simulink model "lpv_modeling_compact"  (R2022b)
settings: Solver=VariableStepAuto  StartTime=0.0  StopTime=25  RelTol=1e-3
values from neighbouring files (symbols this model uses):
  B = [0;0;1]    [coop_lpv.m]    (also in graph_def.m = [1;1;1;1]; lpv_cooperative_control_auto.m; lpv_cooperative_control_man.m)
  C = [1 1 1]    [coop_lpv.m]    (also in lpv_cooperative_control_auto.m; lpv_cooperative_control_man.m)
  D = [0 ;0; 0]    [coop_lpv.m]    (also in graph_def.m = diag(L0); lpv_cooperative_control_auto.m = [0;0;0]; lpv_cooperative_control_man.m = [0;0;0])
  K0 = value(Y0)*inv(value(X))    [lpv_cooperative_control_auto.m]    (also in lpv_cooperative_control_man.m = K_max + theta_max/(theta_max - theta_min)*K_min - theta_max/)
  K1 = value(Y1)*inv(value(X))    [lpv_cooperative_control_auto.m]    (also in lpv_cooperative_control_man.m = K_max/(theta_max - theta_min) - K_min/(theta_max - theta_min)
libraries: cstblocks x4
settings Model: Creator=phatdo  LastModifiedBy=phatdo

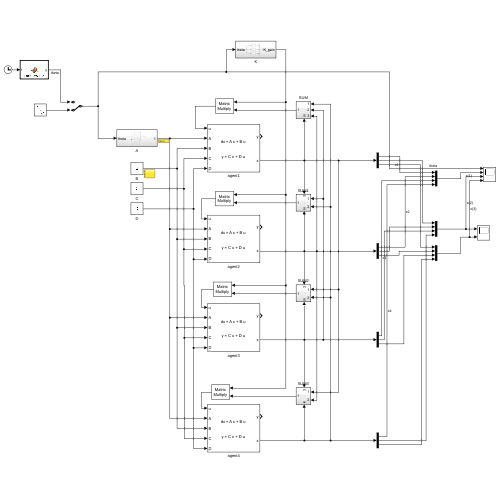
[thumbnail: Simulink's stored preview of the top-level diagram]
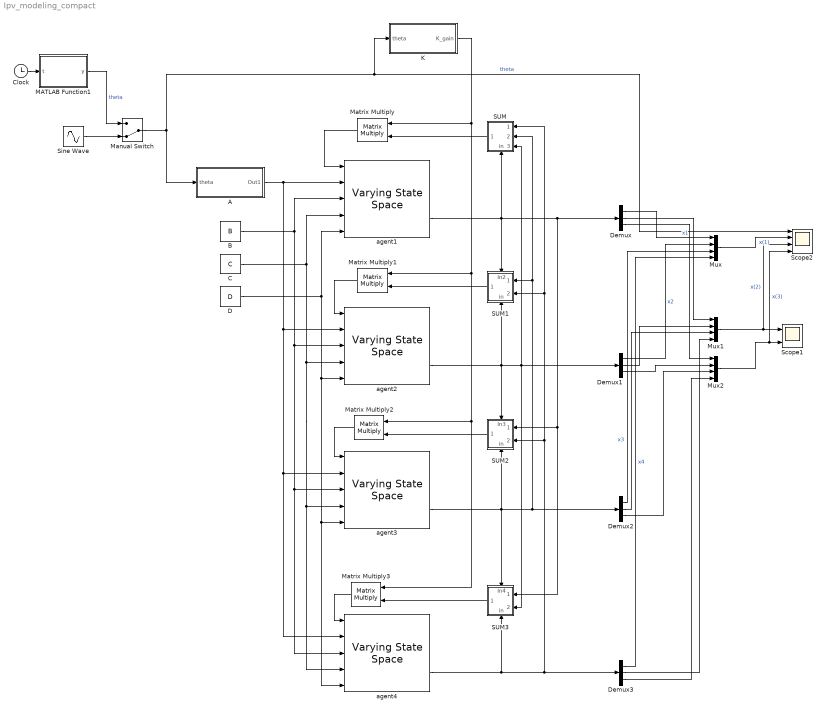
== system lpv_modeling_compact ==
  A : Subsystem
  B : Constant  Value=B
  C : Constant  Value=C  VectorParams1D=off
  Clock : Clock
  D : Constant  Value=D  VectorParams1D=off
  Demux{,1..3} (4 alike) : Demux  Outputs=3
  K : Subsystem
  MATLAB Function1 : MATLAB Function  TreatAsAtomicUnit=on
  Manual Switch : ManualSwitch  CurrentSetting=0
  Matrix Multiply{,1..3} (4 alike) : Product  Multiplication=Matrix(*)
  Mux : Mux
  Mux1 : Mux
  Mux2 : Mux
  SUM : Subsystem
      settings: PortSchema="{\"entries\":[{\"content\":{\"sides\":[{\"content\":{\"connectorIds\":[\"In1\",\"In2\",\"In3\"]},\"type\":\"ConnectorPlacement.EquallySpacedRectSide\",\"uuid\":\"fd34f642-52c8-46e7-b483-8376a438fe66\"},{\"content\":{\"connectorIds\":[\"Out1\"],\"side\":\"RIGHT\"},\"type\":\"ConnectorPlacement.EquallySpacedRectSide\",\"uuid\":\"dec59217-61bd-4aab-963d-2963be1a00c7\"},{\"content\":{\"connectorIds\":[],\"side\":\"TOP\"},\"type\":\"ConnectorPlacement.EquallySpacedRectSide\",\"uuid\":\"ad186b4c-cbd3-48c5-96df-e457cdb7fc4b\"},{\"content\":{\"connectorIds\":[\"In4\"],\"side\":\"BOTTOM\"},\"type\":\"ConnectorPlacement.EquallySpacedRectSide\",\"uuid\":\"5c94262a-f8a6-490c-bbcf-ff9d903d64fd\"}]},\"type\":\"ConnectorPlacement.EquallySpacedConnector\",\"uuid\":\"0cd37f9c-6610-4f40-8695-26be4f4b0f20\"}],\"packageUris\":[\"http://schema.mathworks.com/mf0/Connector/R2020b\"],\"version\":\"1.0\"}"
  SUM1 : Subsystem
      settings: PortSchema="{\"entries\":[{\"content\":{\"sides\":[{\"content\":{\"connectorIds\":[\"In1\",\"In2\"]},\"type\":\"ConnectorPlacement.EquallySpacedRectSide\",\"uuid\":\"fd34f642-52c8-46e7-b483-8376a438fe66\"},{\"content\":{\"connectorIds\":[\"Out1\"],\"side\":\"RIGHT\"},\"type\":\"ConnectorPlacement.EquallySpacedRectSide\",\"uuid\":\"dec59217-61bd-4aab-963d-2963be1a00c7\"},{\"content\":{\"connectorIds\":[\"In3\"],\"side\":\"TOP\"},\"type\":\"ConnectorPlacement.EquallySpacedRectSide\",\"uuid\":\"ad186b4c-cbd3-48c5-96df-e457cdb7fc4b\"},{\"content\":{\"connectorIds\":[\"In4\"],\"side\":\"BOTTOM\"},\"type\":\"ConnectorPlacement.EquallySpacedRectSide\",\"uuid\":\"67af91ab-fe79-430a-80ec-5e8b5dd21872\"}]},\"type\":\"ConnectorPlacement.EquallySpacedConnector\",\"uuid\":\"0cd37f9c-6610-4f40-8695-26be4f4b0f20\"}],\"packageUris\":[\"http://schema.mathworks.com/mf0/Connector/R2020b\"],\"version\":\"1.0\"}"
  SUM2 : Subsystem
      settings: PortSchema="{\"entries\":[{\"content\":{\"sides\":[{\"content\":{\"connectorIds\":[\"In1\",\"In2\"]},\"type\":\"ConnectorPlacement.EquallySpacedRectSide\",\"uuid\":\"fd34f642-52c8-46e7-b483-8376a438fe66\"},{\"content\":{\"connectorIds\":[\"Out1\"],\"side\":\"RIGHT\"},\"type\":\"ConnectorPlacement.EquallySpacedRectSide\",\"uuid\":\"dec59217-61bd-4aab-963d-2963be1a00c7\"},{\"content\":{\"connectorIds\":[\"In3\"],\"side\":\"TOP\"},\"type\":\"ConnectorPlacement.EquallySpacedRectSide\",\"uuid\":\"ad186b4c-cbd3-48c5-96df-e457cdb7fc4b\"},{\"content\":{\"connectorIds\":[\"In4\"],\"side\":\"BOTTOM\"},\"type\":\"ConnectorPlacement.EquallySpacedRectSide\",\"uuid\":\"5210531a-3471-4c70-b5b2-3cd9230d9329\"}]},\"type\":\"ConnectorPlacement.EquallySpacedConnector\",\"uuid\":\"0cd37f9c-6610-4f40-8695-26be4f4b0f20\"}],\"packageUris\":[\"http://schema.mathworks.com/mf0/Connector/R2020b\"],\"version\":\"1.0\"}"
  SUM3 : Subsystem
      settings: PortSchema="{\"entries\":[{\"content\":{\"sides\":[{\"content\":{\"connectorIds\":[\"In1\",\"In2\"]},\"type\":\"ConnectorPlacement.EquallySpacedRectSide\",\"uuid\":\"fd34f642-52c8-46e7-b483-8376a438fe66\"},{\"content\":{\"connectorIds\":[\"Out1\"],\"side\":\"RIGHT\"},\"type\":\"ConnectorPlacement.EquallySpacedRectSide\",\"uuid\":\"dec59217-61bd-4aab-963d-2963be1a00c7\"},{\"content\":{\"connectorIds\":[\"In3\"],\"side\":\"TOP\"},\"type\":\"ConnectorPlacement.EquallySpacedRectSide\",\"uuid\":\"ad186b4c-cbd3-48c5-96df-e457cdb7fc4b\"},{\"content\":{\"connectorIds\":[\"In4\"],\"side\":\"BOTTOM\"},\"type\":\"ConnectorPlacement.EquallySpacedRectSide\",\"uuid\":\"2ed431c9-bcc5-48d0-b09c-89e6b317baf5\"}]},\"type\":\"ConnectorPlacement.EquallySpacedConnector\",\"uuid\":\"0cd37f9c-6610-4f40-8695-26be4f4b0f20\"}],\"packageUris\":[\"http://schema.mathworks.com/mf0/Connector/R2020b\"],\"version\":\"1.0\"}"
  Scope1 : Scope  NumInputPorts=2
  Scope2 : Scope  NumInputPorts=4
  Sine Wave : Sin  Amplitude=0.5  SampleTime=0
  agent1 : cstblocks/Linear Parameter Varying/Varying State Space  x0=[2;0;0]  xNames=''  OutputX=on  OutputDX=off
  agent2 : cstblocks/Linear Parameter Varying/Varying State Space  x0=[0.5;0;0]  xNames=''  OutputX=on  OutputDX=off
  agent3 : cstblocks/Linear Parameter Varying/Varying State Space  x0=[-0.2;0;0]  xNames=''  OutputX=on  OutputDX=off
  agent4 : cstblocks/Linear Parameter Varying/Varying State Space  x0=[-1.8;0;0]  xNames=''  OutputX=on  OutputDX=off
  wires:
  Clock/1 -> MATLAB Function1/1(t)
  Manual Switch/1 -> Scope2/1, K/1(theta), A/1(theta)  "theta"
  C/1 -> agent4/4, agent3/4, agent2/4, agent1/4
  B/1 -> agent4/3, agent3/3, agent2/3, agent1/3
  D/1 -> agent1/5, agent4/5, agent3/5, agent2/5
  A/1(Out1) -> agent4/2, agent3/2, agent2/2, agent1/2
  Matrix Multiply/1 -> agent1/1
  Matrix Multiply1/1 -> agent2/1
  Matrix Multiply2/1 -> agent3/1
  Matrix Multiply3/1 -> agent4/1
  Demux/1 -> Mux/1  "x1"
  Demux1/1 -> Mux/2  "x2"
  Demux2/1 -> Mux/3  "x3"
  Demux3/1 -> Mux/4  "x4"
  Mux/1 -> Scope2/2  "x(1)"
  SUM/1(Out1) -> Matrix Multiply/2
  SUM1/1(Out1) -> Matrix Multiply1/2
  SUM2/1(Out1) -> Matrix Multiply2/2
  SUM3/1(Out1) -> Matrix Multiply3/2
  K/1(K_gain) -> Matrix Multiply/1, Matrix Multiply1/1, Matrix Multiply2/1, Matrix Multiply3/1
  agent1/2 -> SUM2/1(In2), SUM3/1(In2), Demux/1, SUM1/3(In2), SUM/4(in)
  agent2/2 -> SUM/3(In2), Demux1/1, SUM3/2(In3), SUM2/3(In3), SUM1/4(in)
  agent3/2 -> SUM1/1(In4), SUM/2(In4), Demux2/1, SUM3/3(In4), SUM2/4(in)
  agent4/2 -> SUM3/4(in), SUM2/2(In4), SUM1/2(In3), SUM/1(In3), Demux3/1
  MATLAB Function1/1(y) -> Manual Switch/1  "theta"
  Sine Wave/1 -> Manual Switch/2
  Demux/2 -> Mux1/1
  Demux1/2 -> Mux1/2
  Demux2/2 -> Mux1/3
  Demux3/2 -> Mux1/4
  Mux1/1 -> Scope2/3, Scope1/1  "x(2)"
  Demux/3 -> Mux2/1
  Demux1/3 -> Mux2/2
  Demux2/3 -> Mux2/3
  Demux3/3 -> Mux2/4
  Mux2/1 -> Scope2/4, Scope1/2  "x(3)"

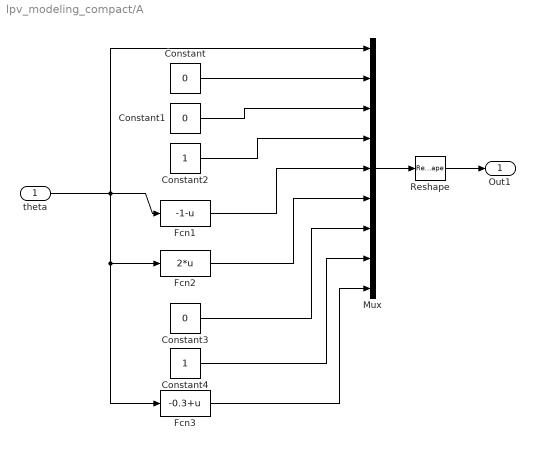
== system lpv_modeling_compact/A ==
  theta : Inport
  Constant : Constant  Value=0
  Constant1 : Constant  Value=0
  Constant2 : Constant
  Constant3 : Constant  Value=0
  Constant4 : Constant
  Fcn1 : Fcn  Expr=-1-u
  Fcn2 : Fcn  Expr=2*u
  Fcn3 : Fcn  Expr=-0.3+u
  Mux : Mux  Inputs=9
  Reshape : Reshape  OutputDimensionality=Customize  OutputDimensions=[3,3]
  Out1 : Outport
  wires:
  Mux/1 -> Reshape/1
  theta/1 -> Fcn3/1, Fcn2/1, Fcn1/1, Mux/1
  Constant/1 -> Mux/2
  Constant1/1 -> Mux/3
  Constant2/1 -> Mux/4
  Fcn1/1 -> Mux/5
  Fcn2/1 -> Mux/6
  Constant3/1 -> Mux/7
  Constant4/1 -> Mux/8
  Reshape/1 -> Out1/1
  Fcn3/1 -> Mux/9

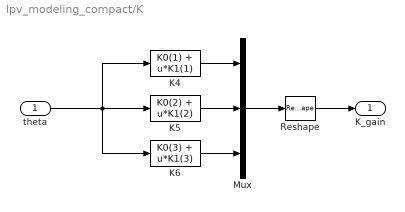
== system lpv_modeling_compact/K ==
  theta : Inport
  K4 : Fcn  Expr=K0(1) + u*K1(1)
  K5 : Fcn  Expr=K0(2) + u*K1(2)
  K6 : Fcn  Expr=K0(3) + u*K1(3)
  Mux : Mux  Inputs=3
  Reshape : Reshape  OutputDimensionality=Customize  OutputDimensions=[1,3]
  K_gain : Outport
  wires:
  Mux/1 -> Reshape/1
  Reshape/1 -> K_gain/1
  K4/1 -> Mux/1
  K5/1 -> Mux/2
  K6/1 -> Mux/3
  theta/1 -> K5/1, K6/1, K4/1

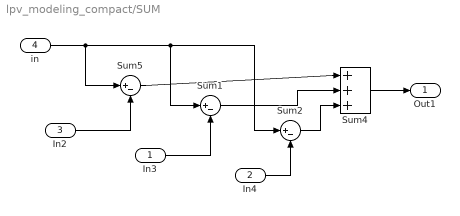
== system lpv_modeling_compact/SUM ==
  In3 : Inport
  In4 : Inport  Port=2
  In2 : Inport  Port=3
  in : Inport  Port=4
  Sum1 : Sum  Inputs=|+-
  Sum2 : Sum  Inputs=|+-
  Sum4 : Sum  Inputs=|+++
  Sum5 : Sum  Inputs=|+-
  Out1 : Outport
  wires:
  in/1 -> Sum5/1, Sum1/1, Sum2/1
  In2/1 -> Sum5/2
  In3/1 -> Sum1/2
  In4/1 -> Sum2/2
  Sum5/1 -> Sum4/1
  Sum1/1 -> Sum4/2
  Sum2/1 -> Sum4/3
  Sum4/1 -> Out1/1

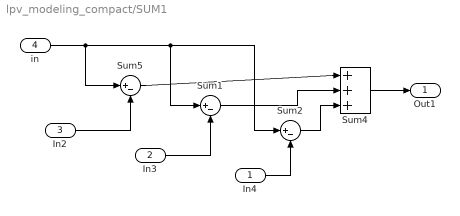
== system lpv_modeling_compact/SUM1 ==
  In4 : Inport
  In3 : Inport  Port=2
  In2 : Inport  Port=3
  in : Inport  Port=4
  Sum1 : Sum  Inputs=|+-
  Sum2 : Sum  Inputs=|+-
  Sum4 : Sum  Inputs=|+++
  Sum5 : Sum  Inputs=|+-
  Out1 : Outport
  wires:
  in/1 -> Sum5/1, Sum1/1, Sum2/1
  In2/1 -> Sum5/2
  In3/1 -> Sum1/2
  In4/1 -> Sum2/2
  Sum5/1 -> Sum4/1
  Sum1/1 -> Sum4/2
  Sum2/1 -> Sum4/3
  Sum4/1 -> Out1/1

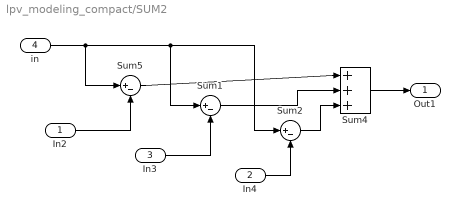
== system lpv_modeling_compact/SUM2 ==
  In2 : Inport
  In4 : Inport  Port=2
  In3 : Inport  Port=3
  in : Inport  Port=4
  Sum1 : Sum  Inputs=|+-
  Sum2 : Sum  Inputs=|+-
  Sum4 : Sum  Inputs=|+++
  Sum5 : Sum  Inputs=|+-
  Out1 : Outport
  wires:
  in/1 -> Sum5/1, Sum1/1, Sum2/1
  In2/1 -> Sum5/2
  In3/1 -> Sum1/2
  In4/1 -> Sum2/2
  Sum5/1 -> Sum4/1
  Sum1/1 -> Sum4/2
  Sum2/1 -> Sum4/3
  Sum4/1 -> Out1/1

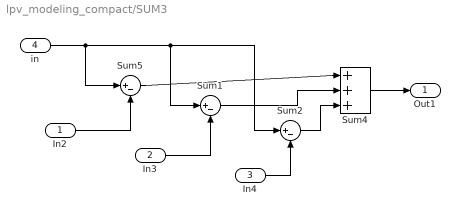
== system lpv_modeling_compact/SUM3 ==
  In2 : Inport
  In3 : Inport  Port=2
  In4 : Inport  Port=3
  in : Inport  Port=4
  Sum1 : Sum  Inputs=|+-
  Sum2 : Sum  Inputs=|+-
  Sum4 : Sum  Inputs=|+++
  Sum5 : Sum  Inputs=|+-
  Out1 : Outport
  wires:
  in/1 -> Sum5/1, Sum1/1, Sum2/1
  In2/1 -> Sum5/2
  In3/1 -> Sum1/2
  In4/1 -> Sum2/2
  Sum5/1 -> Sum4/1
  Sum1/1 -> Sum4/2
  Sum2/1 -> Sum4/3
  Sum4/1 -> Out1/1

== matlab function lpv_modeling_compact/MATLAB Function1 ==
  data: t input; y output
function y = piecewise(t)

if t <= 2
    y = 1.5;
elseif (t > 2) && (t <= 3)
    y = -1;
elseif (t > 3) && (t <= 5)
    y = 1.8;
elseif (t > 5) && (t <= 7)
    y = 0;
elseif (t > 7) && (t <= 9)
    y = 1.1;
else 
    y = -1.2;
end
